simulink model "check"  (R2024a)
settings: Solver=FixedStepAuto  StartTime=0.0  StopTime=10.0  FixedStep=1e-3  RelTol=1e-3
settings Model: Creator=alexe  LastModifiedBy=alexe

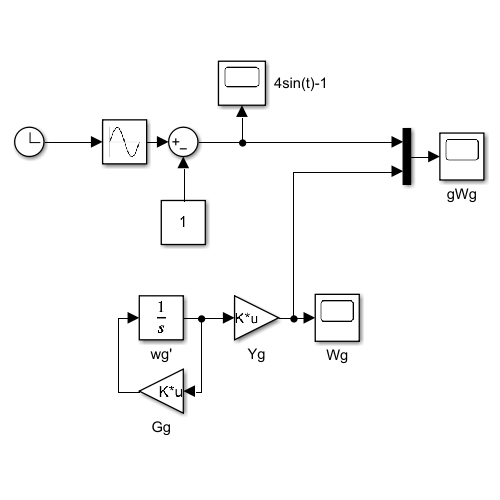
[thumbnail: Simulink's stored preview of the top-level diagram]
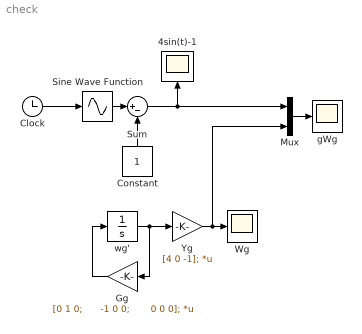
== system check ==
  4sin(t)-1 : Scope
  Clock : Clock
  Constant : Constant
  Gg : Gain  Gain=|  Multiplication=Matrix(K*u)
      | [0 1 0;
      |      -1 0 0;
      |       0 0 0];
  Mux : Mux  Inputs=2
  Sine Wave Function : Sin  TimeSource=Use external signal  Amplitude=4  SampleTime=0
  Sum : Sum  Inputs=|+-
  Wg : Scope
  Yg : Gain  Gain=[4 0 -1];  Multiplication=Matrix(K*u)
  gWg : Scope
  wg' : Integrator  InitialCondition=[0; 1; 1];
  wires:
  Gg/1 -> wg'/1
  wg'/1 -> Gg/1, Yg/1
  Yg/1 -> Mux/2, Wg/1
  Clock/1 -> Sine Wave Function/1
  Sine Wave Function/1 -> Sum/1
  Constant/1 -> Sum/2
  Sum/1 -> Mux/1, 4sin(t)-1/1
  Mux/1 -> gWg/1
